simulink model "q4"  (R2023a)
settings: Solver=VariableStepAuto  StartTime=0.0  StopTime=70  RelTol=1e-3
libraries: simulink x2, commdigbbndam3 x2, commchan3 x1, dspsnks4 x1, commsink2 x1, dspvision x1
settings Model: Creator=giri0  LastModifiedBy=admin

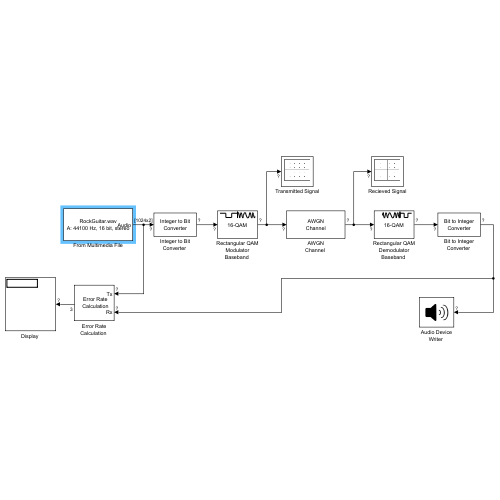
[thumbnail: Simulink's stored preview of the top-level diagram]
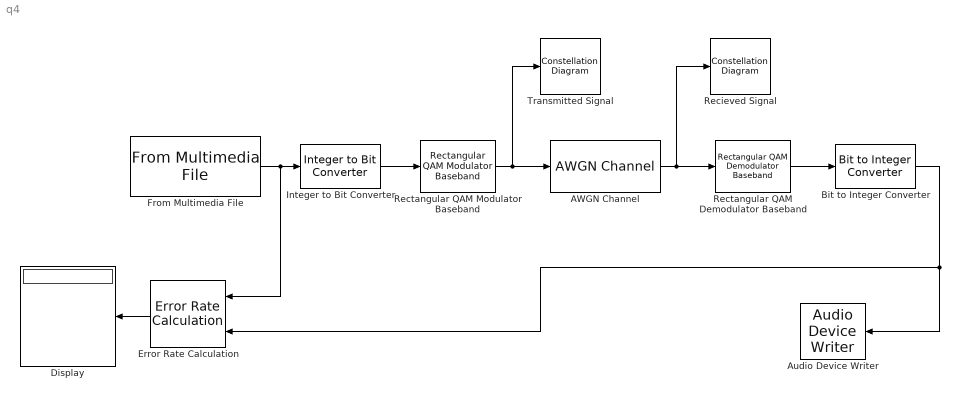
== system q4 ==
  "AWGN Channel " : commchan3/AWGN Channel  LegacyMode=off  NoiseMethod="Signal to noise ratio  (SNR)"  noiseMode="Signal to noise ratio  (SNR)"  EbNo=1e-6  EsNo=10  SNR=20  BitsPerSymbol=4  SignalPower=1  SamplesPerSymbol=1  SymbolPeriod=1  VarianceSource=Parameter  Variance=1  RandomStream=Global stream  Seed=67  SimulateUsing=Code generation
  "Audio Device Writer " : dspsnks4/Audio Device Writer  Driver=DirectSound  Device=Speakers (Realtek(R) Audio)  InheritSampleRate=on  SampleRate=44100  BitDepth=16-bit integer  BufferSize=4096  NumBuffers=10  DefaultOutputChannelMapping=on  OutputChannelMapping=1:2  OutputNumUnderrunSamples=off  DriverIdx=1  DeviceWarnFlag=''
  "Bit to Integer Converter " : simulink/Logic and Bit Operations/Bit to Integer Converter  nbits=16  bitOrder=MSB first  signedOutputValues=Unsigned  outDtype=Inherit via internal rule  outDtypeSigned=Inherit via internal rule
  "Display " : Display
  "Error Rate Calculation " : commsink2/Error Rate Calculation  N=0  st_delay=0  cp_mode=Entire frame  subframe=[]  PMode=Port  WsName=ErrorVec  RsMode2=off  stop=off  numErr=100  maxBits=1e6
  From Multimedia File : dspvision/From Multimedia File  inputFilename=C:\Program Files\MATLAB\R2023a\toolbox\dsp\samples\RockGuitar.wav  readRange=[1 Inf]  loop=on  numPlays=inf  outputStreams=Audio only  videoDataType=single  audioDataType=double  inheritSampleTime=on  userDefinedSampleTime=1/30  noAudioOutput=off  isIntensityVideo=off  fourcc=RGB  colorVideoFormat=Separate color signals  outputEOF=off  dataOrg=Column-major  audioFrameSize=1024  computeAudioFrameSize=off  outSamplingMode=Sample based
      settings: LibrarySourceBlock=dspsrcs4/From Multimedia File
  "Integer to Bit Converter " : simulink/Logic and Bit Operations/Integer to Bit Converter  nbits=16  signedInputValues=Unsigned  bitOrder=MSB first  outDtype=Inherit via internal rule
  Recieved Signal : ConstellationDiagram  WindowPosition=[382.000000,84.000000,600.000000,600.000000,]  ScopeFrameLocation=window
  "Rectangular QAM Demodulator Baseband " : commdigbbndam3/Rectangular QAM Demodulator Baseband  M=16  OutType=Integer  DecType=Hard decision  VarSource=Dialog  Variance=1  Dec=Gray  Mapping=[0:15]  PowType=Peak Power  MinDist=2  AvgPow=1  PeakPow=1  Ph=0  outDtype1=Inherit via internal rule  outDtype2=Inherit via internal rule  derotateFactorWordLen=16  derotateFactorDataTypeStr=Inherit: Same word length as input  derotateFactorLastDataTypeStr=Inherit: Same word length as input  denormFactorWordLen=16  denormFactorDataTypeStr=Inherit: Same word length as input  denormFactorLastDataTypeStr=Inherit: Same word length as input  prodOutWordLen=32  prodOutOverflowMode=Wrap  prodOutRoundingMode=Floor  prodOutOvFlMode=off  prodOutOvFlModeLastStrValue=off  sumWordLen=32
  "Rectangular QAM Modulator Baseband " : commdigbbndam3/Rectangular QAM Modulator Baseband  M=16  InType=Integer  Enc=Gray  Mapping=[0:15]  PowType=Peak Power  MinDist=2  AvgPow=1  PeakPow=1  Ph=0  outDtype=double  outWordLen=16  outUDDataType=sfix(16)  outFracLenMode=Best precision  outFracLen=15  outDataTypeStr=double  outLastDataTypeStr=double
      settings: LibrarySourceBlock=|
      | commhdldigbbndam/Rectangular QAM
      | Modulator
      | Baseband
  Transmitted Signal : ConstellationDiagram  WindowPosition=[391.000000,41.000000,600.000000,600.000000,]  ScopeFrameLocation=window
  wires:
  "AWGN Channel "/1 -> "Rectangular QAM Demodulator Baseband "/1, Recieved Signal/1
  "Error Rate Calculation "/1 -> "Display "/1
  "Rectangular QAM Modulator Baseband "/1 -> Transmitted Signal/1, "AWGN Channel "/1
  "Rectangular QAM Demodulator Baseband "/1 -> "Bit to Integer Converter "/1
  From Multimedia File/1 -> "Error Rate Calculation "/1, "Integer to Bit Converter "/1
  "Integer to Bit Converter "/1 -> "Rectangular QAM Modulator Baseband "/1
  "Bit to Integer Converter "/1 -> "Audio Device Writer "/1, "Error Rate Calculation "/2
